simulink model "DoorLockCntr"  (R2021a)
settings: Solver=FixedStepDiscrete  StartTime=0.0  StopTime=10.0  FixedStep=0.1  RelTol=1e-3  EnableMultiTasking=on
values from neighbouring files (symbols this model uses):
  LockStatus : value not decoded    [DoorLockCntr_data.sldd]
  SpeedCntVal = 20.0    [DoorLockCntr_data.sldd]
  SpeedTh = 5.0    [DoorLockCntr_data.sldd]
libraries: simulink x5
settings Model: DataDictionary=DoorLockCntr_data.sldd  EnableAccessToBaseWorkspace=off  Creator=yyamamot  LastModifiedBy=shayashi
settings SolverCC: AlgebraicLoopSolver=TrustRegion
settings DataIOCC: LimitDataPoints=on  DSMLogging=off  ReturnWorkspaceOutputs=off
settings OptimizationCC: UseFloatMulNetSlope=on  UseSpecifiedMinMax=on  PassReuseOutputArgsAs=Individual arguments  ZeroExternalMemoryAtStartup=off  ZeroInternalMemoryAtStartup=off  NoFixptDivByZeroProtection=on  EfficientFloat2IntCast=on  LifeSpan=1  EfficientTunableParamExpr=on
settings DebuggingCC: SignalRangeChecking=warning  SFUnexpectedBacktrackingDiag=warning  SFNoUnconditionalDefaultTransitionDiag=warning  SFExecutionAtInitializationDiag=none  SFMachineParentedDataDiag=warning  ArithmeticOperatorsInVariantConditions=warning
settings HardwareCC: ProdBitPerSizeT=32  ProdBitPerPtrDiffT=32  ProdWordSize=32  ProdHWDeviceType=Specified
settings ModelReferenceCC: ModelReferenceNumInstancesAllowed=Single  PropagateSignalLabelsOutOfModel=off
settings SFSimCC: SimUseLocalCustomCode=off  MATLABDynamicMemAlloc=off  CustomCodeUndefinedFunction=UseInterfaceOnly
settings RTWCC: SystemTargetFile=ert.tlc  TemplateMakefile=ert_default_tmf  GenerateReport=on  RTWVerbose=off  RTWUseLocalCustomCode=off  BuildConfiguration=Faster Runs  IncludeHyperlinkInReport=on  PortableWordSizes=on  GenerateTraceInfo=on  GenerateTraceReportSl=on  GenerateWebview=on  GenerateCodeMetricsReport=on
settings CodeAppCC: IgnoreCustomStorageClasses=off  StateflowObjectComments=on  ReqsInCode=on
settings ERTTargetCC: MultiwordLength=2048  InferredTypesCompatibility=on  GenerateSampleERTMain=on  IncludeMdlTerminateFcn=off  SuppressErrorStatus=on  SupportAbsoluteTime=off  SupportNonFinite=off  SupportComplex=off  ERTCustomFileTemplate=example_file_process.tlc  MemSecPackage=Simulink
settings ConfigComp: CovMetricSettings=dcmsw  CovHTMLOptions=-sRT=1 -sVT=0 -aTS=1 -bRG=1 -bTC=1 -hTR=0 -nFC=0 -scm=1 -bcm=1 -xEv=0  CovSaveCumulativeToWorkspaceVar=on  CovSaveSingleToWorkspaceVar=on  CovExternalEMLEnable=off  DVSubSystemToStub=1.86070363272185e-315  DVParameterNames=1.86070363272185e-315  DVParameterConstraints=1.86070363272185e-315  DVParameterUseInAnalysis=1.86070363272185e-315  DVModelCoverageObjectives=MCDC  DVMaxTestCaseSteps=500  DVTestSuiteOptimization=LongTestcases  DVDetectDeadLogic=on

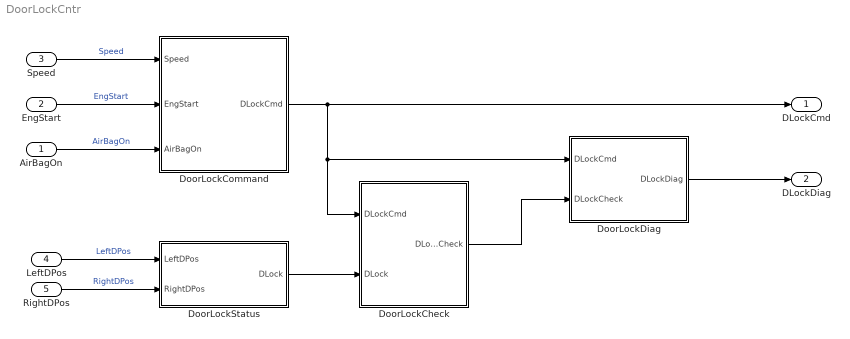
== system DoorLockCntr ==
  AirBagOn : Inport  OutDataTypeStr=boolean  PortDimensions=1  SampleTime=0.1
  EngStart : Inport  Port=2  OutDataTypeStr=boolean  PortDimensions=1  SampleTime=0.1
  Speed : Inport  Port=3  OutDataTypeStr=single  PortDimensions=1  SampleTime=0.1
  LeftDPos : Inport  Port=4  OutDataTypeStr=single  PortDimensions=1  SampleTime=0.1
  RightDPos : Inport  Port=5  OutDataTypeStr=single  PortDimensions=1  SampleTime=0.1
  DoorLockCheck : Subsystem  TreatAsAtomicUnit=on
      settings: RTWSystemCode=Nonreusable function  RTWFcnNameOpts=Use subsystem name
  DoorLockCommand : Subsystem  TreatAsAtomicUnit=on
      settings: RTWSystemCode=Nonreusable function  RTWFcnNameOpts=Use subsystem name
  DoorLockDiag : Subsystem  TreatAsAtomicUnit=on
      settings: RTWSystemCode=Nonreusable function  RTWFcnNameOpts=Use subsystem name
  DoorLockStatus : Subsystem  TreatAsAtomicUnit=on
      settings: RTWSystemCode=Nonreusable function  RTWFcnNameOpts=Use subsystem name
  DLockCmd : Outport
  DLockDiag : Outport  Port=2
  wires:
  Speed/1 -> DoorLockCommand/1(Speed)  "Speed"
  EngStart/1 -> DoorLockCommand/2(EngStart)  "EngStart"
  AirBagOn/1 -> DoorLockCommand/3(AirBagOn)  "AirBagOn"
  LeftDPos/1 -> DoorLockStatus/1(LeftDPos)  "LeftDPos"
  RightDPos/1 -> DoorLockStatus/2(RightDPos)  "RightDPos"
  DoorLockDiag/1(DLockDiag) -> DLockDiag/1
  DoorLockStatus/1(DLock) -> DoorLockCheck/2(DLock)
  DoorLockCheck/1(DLockCheck) -> DoorLockDiag/2(DLockCheck)
  DoorLockCommand/1(DLockCmd) -> DLockCmd/1, DoorLockDiag/1(DLockCmd), DoorLockCheck/1(DLockCmd)

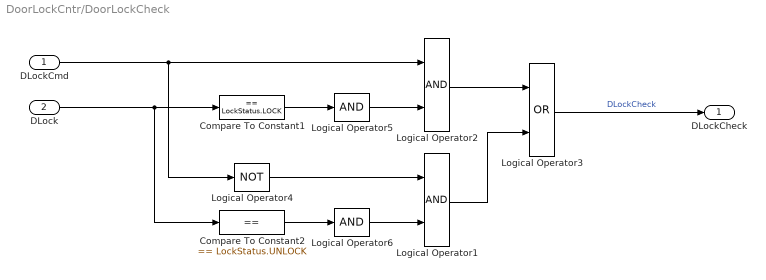
== system DoorLockCntr/DoorLockCheck ==
  DLockCmd : Inport
  DLock : Inport  Port=2
  Compare To Constant1 : simulink/Logic and Bit Operations/Compare To Constant  relop===  const=LockStatus.LOCK  OutDataTypeStr=boolean
  Compare To Constant2 : simulink/Logic and Bit Operations/Compare To Constant  relop===  const=LockStatus.UNLOCK  OutDataTypeStr=boolean
  Logical Operator1 : Logic  AllPortsSameDT=off  OutDataTypeStr=boolean
  Logical Operator2 : Logic  AllPortsSameDT=off  OutDataTypeStr=boolean
  Logical Operator3 : Logic  Operator=OR  AllPortsSameDT=off  OutDataTypeStr=boolean
  Logical Operator4 : Logic  Operator=NOT  AllPortsSameDT=off  OutDataTypeStr=boolean
  Logical Operator5 : Logic  Inputs=1  AllPortsSameDT=off  OutDataTypeStr=boolean
  Logical Operator6 : Logic  Inputs=1  AllPortsSameDT=off  OutDataTypeStr=boolean
  DLockCheck : Outport
  wires:
  DLock/1 -> Compare To Constant1/1, Compare To Constant2/1
  Logical Operator3/1 -> DLockCheck/1  "DLockCheck"
  Logical Operator5/1 -> Logical Operator2/2
  Compare To Constant1/1 -> Logical Operator5/1
  DLockCmd/1 -> Logical Operator4/1, Logical Operator2/1
  Logical Operator6/1 -> Logical Operator1/2
  Compare To Constant2/1 -> Logical Operator6/1
  Logical Operator1/1 -> Logical Operator3/2
  Logical Operator2/1 -> Logical Operator3/1
  Logical Operator4/1 -> Logical Operator1/1

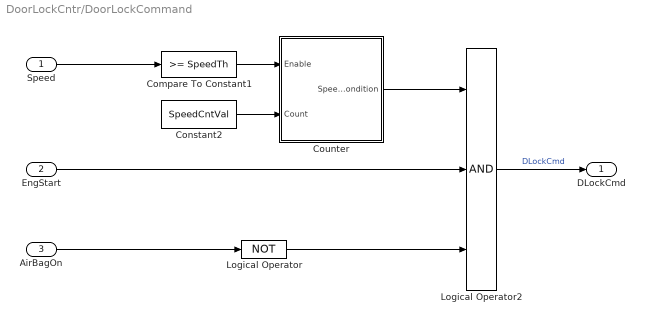
== system DoorLockCntr/DoorLockCommand ==
  Speed : Inport
  EngStart : Inport  Port=2
  AirBagOn : Inport  Port=3  OutDataTypeStr=boolean  PortDimensions=1  SampleTime=[0.10000000000000001,0]
  Compare To Constant1 : simulink/Logic and Bit Operations/Compare To Constant  relop=>=  const=SpeedTh  OutDataTypeStr=boolean
  Constant2 : Constant  Value=SpeedCntVal  OutDataTypeStr=uint8
      settings: AttributesFormatString=DataType = %<OutDataTypeStr>
  Counter : Subsystem
  Logical Operator : Logic  Operator=NOT  AllPortsSameDT=off  OutDataTypeStr=boolean
  Logical Operator2 : Logic  Inputs=3  AllPortsSameDT=off  OutDataTypeStr=boolean
  DLockCmd : Outport
  wires:
  Logical Operator/1 -> Logical Operator2/3
  Constant2/1 -> Counter/2(Count)
  Counter/1(SpeedCondition) -> Logical Operator2/1
  Logical Operator2/1 -> DLockCmd/1  "DLockCmd"
  AirBagOn/1 -> Logical Operator/1
  Compare To Constant1/1 -> Counter/1(Enable)
  EngStart/1 -> Logical Operator2/2
  Speed/1 -> Compare To Constant1/1

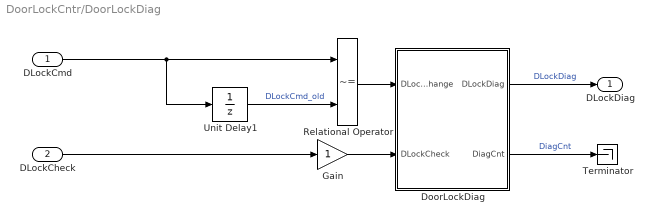
== system DoorLockCntr/DoorLockDiag ==
  DLockCmd : Inport
  DLockCheck : Inport  Port=2
  DoorLockDiag : Stateflow chart  TreatAsAtomicUnit=on
  Gain : Gain
  Relational Operator : RelationalOperator  Operator=~=  OutDataTypeStr=boolean  RndMeth=Nearest
  Terminator : Terminator
  Unit Delay1 : UnitDelay  SampleTime=-1  StateName=DLockCmd_prev  HasFrameUpgradeWarning=on  StateMustResolveToSignalObject=on
      settings: AttributesFormatString=InitialValue = %<InitialCondition>\nState = %<StateName>
  DLockDiag : Outport
  wires:
  DoorLockDiag/2(DiagCnt) -> Terminator/1  "DiagCnt"
  DLockCmd/1 -> Relational Operator/1, Unit Delay1/1
  Unit Delay1/1 -> Relational Operator/2  "DLockCmd_old"
  DoorLockDiag/1(DLockDiag) -> DLockDiag/1  "DLockDiag"
  DLockCheck/1 -> Gain/1
  Relational Operator/1 -> DoorLockDiag/1(DLockCmdChange)
  Gain/1 -> DoorLockDiag/2(DLockCheck)

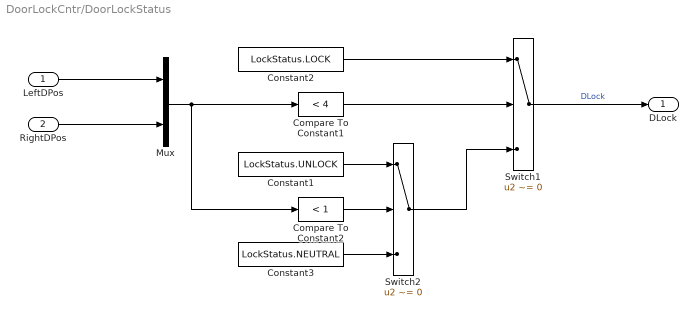
== system DoorLockCntr/DoorLockStatus ==
  LeftDPos : Inport
  RightDPos : Inport  Port=2
  Compare To Constant1 : simulink/Logic and Bit Operations/Compare To Constant  relop=<  const=4  OutDataTypeStr=boolean
  Compare To Constant2 : simulink/Logic and Bit Operations/Compare To Constant  relop=<  const=1  OutDataTypeStr=boolean
  Constant1 : Constant  Value=LockStatus.UNLOCK  OutDataTypeStr=Enum: LockStatus
      settings: AttributesFormatString=DataType = %<OutDataTypeStr>
  Constant2 : Constant  Value=LockStatus.LOCK  OutDataTypeStr=Enum: LockStatus
      settings: AttributesFormatString=DataType = %<OutDataTypeStr>
  Constant3 : Constant  Value=LockStatus.NEUTRAL  OutDataTypeStr=Enum: LockStatus
      settings: AttributesFormatString=DataType = %<OutDataTypeStr>
  Mux : Mux  Inputs=2
  Switch1 : Switch  Criteria=u2 ~= 0  RndMeth=Simplest
  Switch2 : Switch  Criteria=u2 ~= 0  RndMeth=Simplest
  DLock : Outport
  wires:
  Switch1/1 -> DLock/1  "DLock"
  Constant3/1 -> Switch2/3
  Compare To Constant1/1 -> Switch1/2
  RightDPos/1 -> Mux/2
  Constant1/1 -> Switch2/1
  Compare To Constant2/1 -> Switch2/2
  Switch2/1 -> Switch1/3
  LeftDPos/1 -> Mux/1
  Constant2/1 -> Switch1/1
  Mux/1 -> Compare To Constant1/1, Compare To Constant2/1

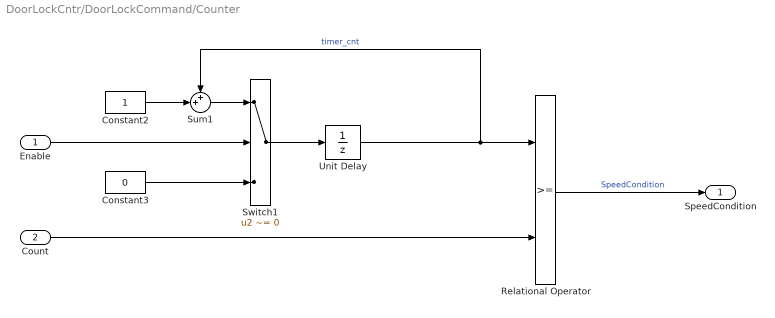
== system DoorLockCntr/DoorLockCommand/Counter ==
  Enable : Inport
  Count : Inport  Port=2
  Constant2 : Constant  OutDataTypeStr=uint8
      settings: AttributesFormatString=DataType = %<OutDataTypeStr>
  Constant3 : Constant  Value=0  OutDataTypeStr=uint8
      settings: AttributesFormatString=DataType = %<OutDataTypeStr>
  Relational Operator : RelationalOperator  OutDataTypeStr=boolean  RndMeth=Nearest
  Sum1 : Sum  Inputs=++|  RndMeth=Simplest
      settings: AttributesFormatString=SatInt = %<SaturateOnIntegerOverflow>
  Switch1 : Switch  Criteria=u2 ~= 0  RndMeth=Simplest
  Unit Delay : UnitDelay  SampleTime=-1  StateName=SpeedCnt  HasFrameUpgradeWarning=on  StateMustResolveToSignalObject=on
      settings: AttributesFormatString=InitialValue = %<InitialCondition>\nState = %<StateName>
  SpeedCondition : Outport
  wires:
  Relational Operator/1 -> SpeedCondition/1  "SpeedCondition"
  Count/1 -> Relational Operator/2
  Constant2/1 -> Sum1/2
  Sum1/1 -> Switch1/1
  Unit Delay/1 -> Sum1/1, Relational Operator/1  "timer_cnt"
  Switch1/1 -> Unit Delay/1
  Constant3/1 -> Switch1/3
  Enable/1 -> Switch1/2

== stateflow chart DoorLockCntr/DoorLockDiag/DoorLockDiag ==
  state NORMAL
    entry:
    DLockDiag = false;
  state WARNING
    entry:
    DiagCnt = 1;
    during:
    DiagCnt++;
  state FAIL
    entry:
    DLockDiag = true;
  (default) -> NORMAL
  NORMAL -> WARNING : [DLockCmdChange]
  (junction 7) -> NORMAL [order 1] : [DLockCheck]
  WARNING -> WARNING [order 1] : [DLockCmdChange]
  WARNING -> (junction 7) [order 2] : [DiagCnt == DiagCntVal]
  (junction 7) -> FAIL [order 2]
  data: DLockCmdChange input; DLockCheck input; DLockDiag output boolean; DiagCntVal parameter; DiagCnt output uint8
